simulink model "Model_z_regulatorem"  (R2024b)
settings: Solver=VariableStepAuto  StartTime=0.0  StopTime=20000  MaxStep=1  RelTol=1e-3
values from neighbouring files (symbols this model uses):
  czas_skok = 1000    [uklad_regulacji.m]
  dPg = 1000    [uklad_regulacji.m]
  dSP = 2    [uklad_regulacji.m]
  K = y_delta/ dPg    [uklad_regulacji.m]
  K_rp = 0.9*T/(K*T_0)    [uklad_regulacji.m]
  SP0 = T_pn    (= 15)    [uklad_regulacji.m]
  T = 1758    [uklad_regulacji.m]
  T_0 = 100    [uklad_regulacji.m]
  T_i = 3.33*T_0    (= 333)    [uklad_regulacji.m]
  T_p0 = (K_p*(T_wewn0)+K_d*T_zewn0)/(K_p+K_d)    (= 15)    [uklad_regulacji.m]
settings Model: Creator=userbrigh  LastModifiedBy=userbrigh

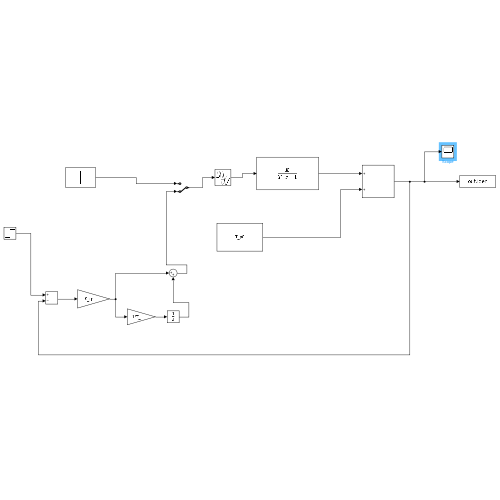
[thumbnail: Simulink's stored preview of the top-level diagram]
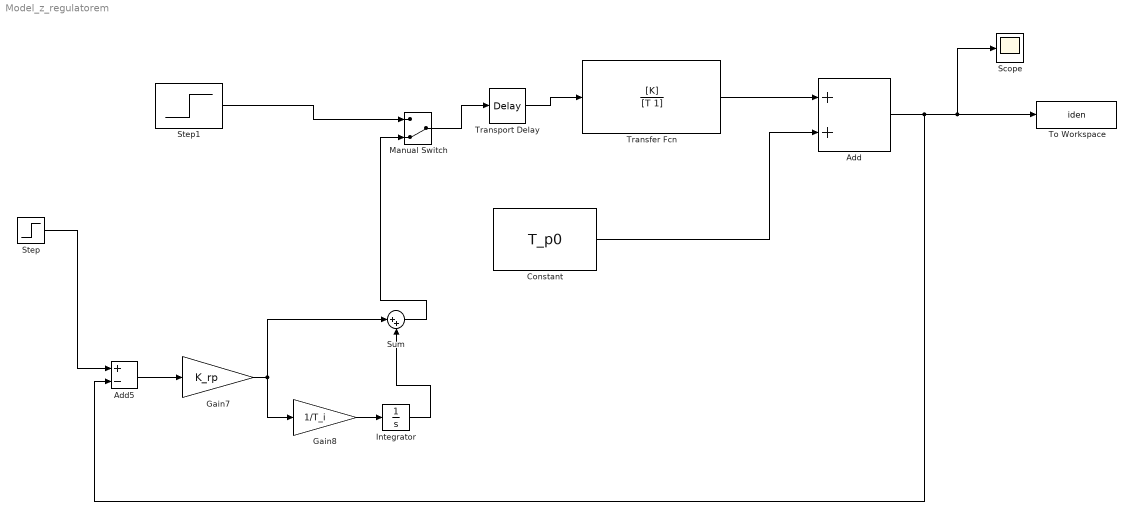
== system Model_z_regulatorem ==
  Add : Sum
  Add5 : Sum  Inputs=+-
  Constant : Constant  Value=T_p0
  Gain7 : Gain  Gain=K_rp
  Gain8 : Gain  Gain=1/T_i
  Integrator : Integrator
  Manual Switch : ManualSwitch  CurrentSetting=0
  Scope : Scope
  Step : Step  Time=czas_skok  Before=SP0  After=SP0+dSP  SampleTime=0
  Step1 : Step  Time=czas_skok  After=dPg  SampleTime=0
  Sum : Sum  Inputs=|++
  To Workspace : ToWorkspace  VariableName=iden  SampleTime=-1
  Transfer Fcn : TransferFcn  Numerator=[K]  Denominator=[T 1]
  Transport Delay : TransportDelay  DelayTime=T_0
  wires:
  Integrator/1 -> Sum/2
  Gain7/1 -> Sum/1, Gain8/1
  Gain8/1 -> Integrator/1
  Add5/1 -> Gain7/1
  Sum/1 -> Manual Switch/2
  Transport Delay/1 -> Transfer Fcn/1
  Add/1 -> Add5/2, To Workspace/1, Scope/1
  Transfer Fcn/1 -> Add/1
  Constant/1 -> Add/2
  Step1/1 -> Manual Switch/1
  Manual Switch/1 -> Transport Delay/1
  Step/1 -> Add5/1
